simulink model "CruiseControl_pp"  (R2018b)
settings: Solver=ode3  StartTime=0.0  StopTime=16  FixedStep=0.1  RelTol=1e-3  EnableMultiTasking=on
PreLoadFcn:
  | CruiseControl_dd;
  | definePPenums;
undefined symbols (not defined in the file or in its folder): mintspeed
libraries: sldvlib x20, simulink x7
settings Model: SnapshotInterval=1  Creator=The MathWorks Inc.  LastModifiedBy=colosky
settings DataIOCC: LimitDataPoints=on  SaveFormat=Array  SaveOutput=off  SaveTime=off
settings OptimizationCC: DefaultParameterBehavior=Inlined  InlineInvariantSignals=on  ExpressionDepthLimit=2147483647  InitFltsAndDblsToZero=on  LifeSpan=1
settings DebuggingCC: SaveWithParameterizedLinksMsg=none  UnderspecifiedInitializationDetection=Classic  MergeDetectMultiDrivingBlocksExec=none  SolverPrmCheckMsg=warning  FcnCallInpInsideContextMsg=warning  AllowSymbolicDim=off  StateNameClashWarn=warning  LibraryContextMissingDiagnostic=none  StrictBusMsg=ErrorOnBusTreatedAsVector  SFUnexpectedBacktrackingDiag=warning  SFNoUnconditionalDefaultTransitionDiag=warning  SFExecutionAtInitializationDiag=none
settings HardwareCC: ProdBitPerPointer=32  ProdBitPerSizeT=32  ProdBitPerPtrDiffT=32  ProdLargestAtomicFloat=None  ProdEndianess=Unspecified  ProdWordSize=32  ProdHWDeviceType=32-bit Generic
settings ModelReferenceCC: ModelReferenceNumInstancesAllowed=Single  PropagateSignalLabelsOutOfModel=off
settings SFSimCC: SimUseLocalCustomCode=off  SimParseCustomCode=off  MATLABDynamicMemAlloc=off
settings RTWCC: SystemTargetFile=ert.tlc  TemplateMakefile=ert_default_tmf  GenerateReport=on  RTWUseLocalCustomCode=off  IncludeHyperlinkInReport=on  LaunchReport=on  GenerateTraceInfo=on  GenerateTraceReport=on  GenerateTraceReportSl=on  GenerateTraceReportSf=on  GenerateTraceReportEml=on
settings CodeAppCC: ForceParamTrailComments=on  IgnoreCustomStorageClasses=off  OperatorAnnotations=on  SimulinkDataObjDesc=on  SFDataObjDesc=on  MATLABFcnDesc=on  InsertBlockDesc=on  StateflowObjectComments=on  MATLABSourceComments=on
settings ERTTargetCC: MultiwordLength=2048  GenerateSampleERTMain=on  InlinedParameterPlacement=NonHierarchical  ERTCustomFileTemplate=example_file_process.tlc
settings ConfigComp: CovEnable=on  CovScope=ReferencedModels  RecordCoverage=on  CovMetricSettings=dcme  CovModelRefEnable=Off  CovExternalEMLEnable=off  CovSFcnEnable=off  DVMode=PropertyProving  DVMaxProcessTime=3000  DVDisplayUnsatisfiableObjectives=on  DVAutomaticStubbing=off  DVMakeOutputFilesUnique=off  DVModelCoverageObjectives=MCDC  DVMaxTestCaseSteps=500  DVTestSuiteOptimization=CombinedObjectives  DVAssertions=EnableAll  DVProofAssumptions=EnableAll  DVDetectActiveLogic=on  DVDetectIntegerOverflow=off  DVMaxViolationSteps=10  DVSaveDataFile=off  DVSaveHarnessModel=on  DVReportIncludeGraphics=on  DVDisplayResultsOnModel=on

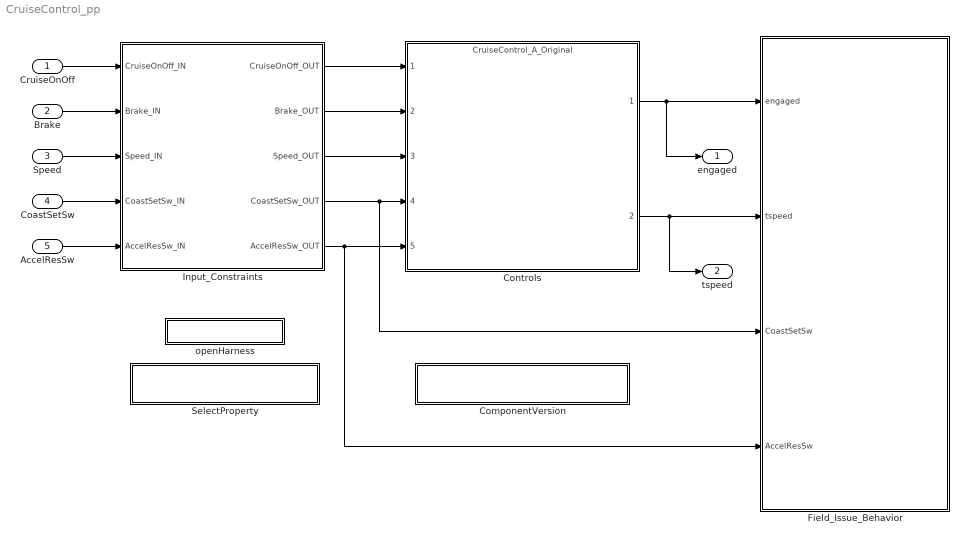
== system CruiseControl_pp ==
  CruiseOnOff : Inport  OutDataTypeStr=boolean  PortDimensions=1
  Brake : Inport  Port=2  OutDataTypeStr=boolean  PortDimensions=1
  Speed : Inport  Port=3  OutDataTypeStr=uint8  PortDimensions=1
  CoastSetSw : Inport  Port=4  OutDataTypeStr=boolean  PortDimensions=1
  AccelResSw : Inport  Port=5  OutDataTypeStr=boolean  PortDimensions=1
  ComponentVersion : Subsystem
      settings: OpenFcn=|
      | [~,enumVers] = enumeration('CtrlsVerEnum');
      | [selection, ok] = listdlg('Name','Component Version','ListSize',[210 110],'SelectionMode','single', ...
      |    'PromptString','Select Cruise Control version...','ListString',enumVers,'InitialValue',uint32(CtrlsVer));
      | waitfor(selection);
      | if ok
      |    CtrlsVer = CtrlsVerEnum(enumVers{selection});
      | end
      mask Display: disp('Select Cruise Control version to verify');
  Controls : ModelReference  ModelNameDialog=CruiseControl_A_Original.slx  SimulationMode=Normal  Variant=on  ModelReferenceVersion=1.516
  Field_Issue_Behavior : Subsystem  Variant=on
      settings: AttributesFormatString=%<BlockChoice>
  Input_Constraints : Subsystem  Variant=on
      settings: AttributesFormatString=%<BlockChoice>
  SelectProperty : Subsystem
      settings: OpenFcn=|
      | [~,enumProps] = enumeration('PropEnum');
      | [selection, ok] = listdlg('Name','Propery To Prove','ListSize',[210 110],'SelectionMode','single', ...
      |    'PromptString','Select Property to Prove...','ListString',enumProps,'InitialValue',uint32(Prop2Prove));
      | waitfor(selection);
      | if ok
      |    Prop2Prove = PropEnum(enumProps{selection});
      | end
      mask Display: disp('Select Property to Prove...');
  openHarness : Subsystem
      settings: OpenFcn=|
      | switch (CtrlsVer)
      | case CtrlsVerEnum.CtrlC_ExecOrder_fix
      |     load_PP_harness('CruiseControl_pp_harness_FieldIssue');
      | case CtrlsVerEnum.CtrlD_ExecOrderSneak_fix
      |     load_PP_harness('CruiseControl_pp_harness_ReqProve');
      | case CtrlsVerEnum.CtrlE_ExecOrderSneakDblReject_fix
      |     load_PP_harness('CruiseControl_pp_harness_ReqWithParsProve');
      | end
      mask Display: disp(['Open Harness']);
  engaged : Outport  OutDataTypeStr=boolean  PortDimensions=1
  tspeed : Outport  Port=2  OutDataTypeStr=uint8  PortDimensions=1
  wires:
  Controls/2 -> tspeed/1, Field_Issue_Behavior/2(tspeed)
  AccelResSw/1 -> Input_Constraints/5(AccelResSw_IN)
  Speed/1 -> Input_Constraints/3(Speed_IN)
  CruiseOnOff/1 -> Input_Constraints/1(CruiseOnOff_IN)
  Brake/1 -> Input_Constraints/2(Brake_IN)
  CoastSetSw/1 -> Input_Constraints/4(CoastSetSw_IN)
  Input_Constraints/1(CruiseOnOff_OUT) -> Controls/1
  Input_Constraints/2(Brake_OUT) -> Controls/2
  Input_Constraints/3(Speed_OUT) -> Controls/3
  Input_Constraints/4(CoastSetSw_OUT) -> Field_Issue_Behavior/3(CoastSetSw), Controls/4
  Input_Constraints/5(AccelResSw_OUT) -> Field_Issue_Behavior/4(AccelResSw), Controls/5
  Controls/1 -> engaged/1, Field_Issue_Behavior/1(engaged)

== system CruiseControl_pp/ComponentVersion ==

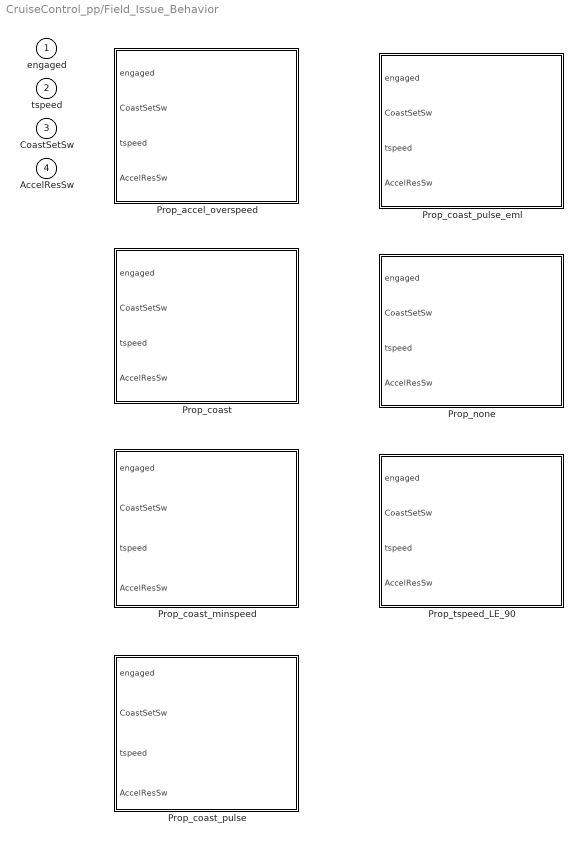
== system CruiseControl_pp/Field_Issue_Behavior ==
  engaged : Inport
  tspeed : Inport  Port=2
  CoastSetSw : Inport  Port=3
  AccelResSw : Inport  Port=4
  Prop_accel_overspeed : Subsystem  VariantControl=Prop2Prove == PropEnum.Prop_accel_overspeed
  Prop_coast : Subsystem  VariantControl=Prop2Prove == PropEnum.Prop_coast
  Prop_coast_minspeed : Subsystem  VariantControl=Prop2Prove == PropEnum.Prop_coast_minspeed
  Prop_coast_pulse : Subsystem  VariantControl=Prop2Prove == PropEnum.Prop_coast_pulse
  Prop_coast_pulse_eml : Subsystem  VariantControl=Prop2Prove == PropEnum.Prop_coast_pulse_eml
  Prop_none : Subsystem  VariantControl=Prop2Prove == PropEnum.Prop_none
  Prop_tspeed_LE_90 : Subsystem  VariantControl=Prop2Prove == PropEnum.Prop_tspeed_LE_90

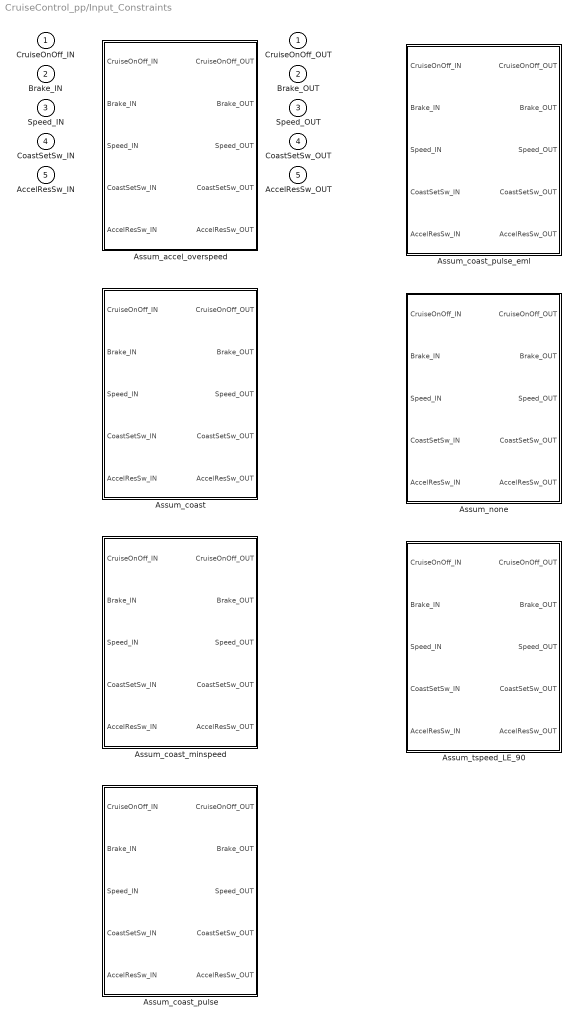
== system CruiseControl_pp/Input_Constraints ==
  CruiseOnOff_IN : Inport
  Brake_IN : Inport  Port=2
  Speed_IN : Inport  Port=3
  CoastSetSw_IN : Inport  Port=4
  AccelResSw_IN : Inport  Port=5
  Assum_accel_overspeed : Subsystem  VariantControl=Prop2Prove == PropEnum.Prop_accel_overspeed
  Assum_coast : Subsystem  VariantControl=Prop2Prove == PropEnum.Prop_coast
  Assum_coast_minspeed : Subsystem  VariantControl=Prop2Prove == PropEnum.Prop_coast_minspeed
  Assum_coast_pulse : Subsystem  VariantControl=Prop2Prove == PropEnum.Prop_coast_pulse
  Assum_coast_pulse_eml : Subsystem  VariantControl=Prop2Prove == PropEnum.Prop_coast_pulse_eml
  Assum_none : Subsystem  VariantControl=Prop2Prove == PropEnum.Prop_none
  Assum_tspeed_LE_90 : Subsystem  VariantControl=Prop2Prove == PropEnum.Prop_tspeed_LE_90
  CruiseOnOff_OUT : Outport
  Brake_OUT : Outport  Port=2
  Speed_OUT : Outport  Port=3
  CoastSetSw_OUT : Outport  Port=4
  AccelResSw_OUT : Outport  Port=5

== system CruiseControl_pp/SelectProperty ==

== system CruiseControl_pp/openHarness ==

== system CruiseControl_pp/Field_Issue_Behavior/Prop_accel_overspeed ==
  engaged : Inport
  CoastSetSw : Inport  Port=2
  tspeed : Inport  Port=3
  AccelResSw : Inport  Port=4
  Compare To Constant : simulink/Logic and Bit Operations/Compare To Constant  relop=<=  const=95  OutDataTypeStr=boolean
  EngagedImplies : sldvlib/Verification Utilities/Implies
      settings: SourceProductName=Simulink Design Verifier  SourceProductBaseCode=DV
  Logical Operator2 : Logic  AllPortsSameDT=off  OutDataTypeStr=boolean
  Prop_accel_overspeed : sldvlib/Objectives and Constraints/Proof Objective  enabled=on  customAVTBlockType=Proof Objective  intervals=true  dispValues=on  outEnabled=off  enableStopSim=off
      settings: AttributesFormatString=%<intervals>  SourceProductName=Simulink Design Verifier  SourceProductBaseCode=DV
  Terminator1 : Terminator
  wires:
  CoastSetSw/1 -> Terminator1/1
  tspeed/1 -> Compare To Constant/1
  Compare To Constant/1 -> EngagedImplies/2
  engaged/1 -> Logical Operator2/1
  AccelResSw/1 -> Logical Operator2/2
  Logical Operator2/1 -> EngagedImplies/1
  EngagedImplies/1 -> Prop_accel_overspeed/1

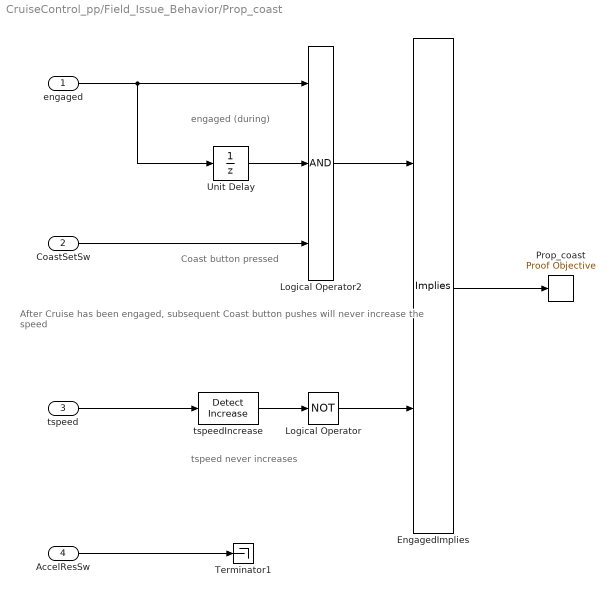
== system CruiseControl_pp/Field_Issue_Behavior/Prop_coast ==
  note: engaged (during)
  note: tspeed never increases
  note: Coast button pressed
  note: After Cruise has been engaged, subsequent Coast button pushes will never increase the speed
  engaged : Inport
  CoastSetSw : Inport  Port=2
  tspeed : Inport  Port=3
  AccelResSw : Inport  Port=4
  EngagedImplies : sldvlib/Verification Utilities/Implies
      settings: SourceProductName=Simulink Design Verifier  SourceProductBaseCode=DV
  Logical Operator : Logic  Operator=NOT  AllPortsSameDT=off  OutDataTypeStr=boolean
  Logical Operator2 : Logic  Inputs=3  AllPortsSameDT=off  OutDataTypeStr=boolean
  Prop_coast : sldvlib/Objectives and Constraints/Proof Objective  enabled=on  customAVTBlockType=Proof Objective  intervals=true  dispValues=on  outEnabled=off  enableStopSim=off
      settings: AttributesFormatString=%<intervals>  SourceProductName=Simulink Design Verifier  SourceProductBaseCode=DV
  Terminator1 : Terminator
  Unit Delay : UnitDelay  SampleTime=-1
  tspeedIncrease : simulink/Logic and Bit Operations/Detect Increase  vinit=0.0  InputProcessing=Inherited  OutDataTypeStr=boolean
  wires:
  Logical Operator2/1 -> EngagedImplies/1
  CoastSetSw/1 -> Logical Operator2/3
  Logical Operator/1 -> EngagedImplies/2
  engaged/1 -> Unit Delay/1, Logical Operator2/1
  AccelResSw/1 -> Terminator1/1
  Unit Delay/1 -> Logical Operator2/2
  tspeed/1 -> tspeedIncrease/1
  tspeedIncrease/1 -> Logical Operator/1
  EngagedImplies/1 -> Prop_coast/1

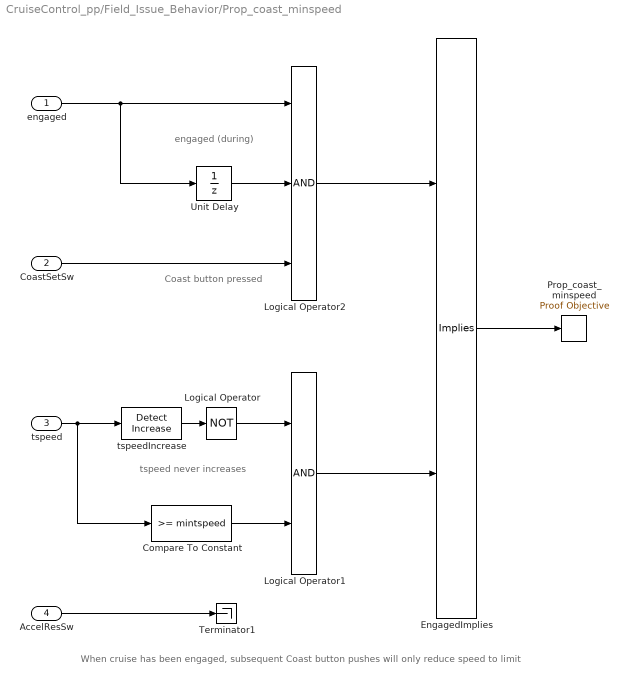
== system CruiseControl_pp/Field_Issue_Behavior/Prop_coast_minspeed ==
  note: engaged (during)
  note: tspeed never increases
  note: Coast button pressed
  note: When cruise has been engaged, subsequent Coast button pushes will only reduce speed to limit
  engaged : Inport
  CoastSetSw : Inport  Port=2
  tspeed : Inport  Port=3
  AccelResSw : Inport  Port=4
  Compare To Constant : simulink/Logic and Bit Operations/Compare To Constant  relop=>=  const=mintspeed  OutDataTypeStr=boolean
  EngagedImplies : sldvlib/Verification Utilities/Implies
      settings: SourceProductName=Simulink Design Verifier  SourceProductBaseCode=DV
  Logical Operator : Logic  Operator=NOT  AllPortsSameDT=off  OutDataTypeStr=boolean
  Logical Operator1 : Logic  AllPortsSameDT=off  OutDataTypeStr=boolean
  Logical Operator2 : Logic  Inputs=3  AllPortsSameDT=off  OutDataTypeStr=boolean
  Prop_coast_minspeed : sldvlib/Objectives and Constraints/Proof Objective  enabled=on  customAVTBlockType=Proof Objective  intervals=true  dispValues=on  outEnabled=off  enableStopSim=off
      settings: AttributesFormatString=%<intervals>  SourceProductName=Simulink Design Verifier  SourceProductBaseCode=DV
  Terminator1 : Terminator
  Unit Delay : UnitDelay  SampleTime=-1
  tspeedIncrease : simulink/Logic and Bit Operations/Detect Increase  vinit=0.0  InputProcessing=Inherited  OutDataTypeStr=boolean
  wires:
  Logical Operator2/1 -> EngagedImplies/1
  CoastSetSw/1 -> Logical Operator2/3
  engaged/1 -> Unit Delay/1, Logical Operator2/1
  AccelResSw/1 -> Terminator1/1
  Unit Delay/1 -> Logical Operator2/2
  tspeed/1 -> Compare To Constant/1, tspeedIncrease/1
  tspeedIncrease/1 -> Logical Operator/1
  EngagedImplies/1 -> Prop_coast_minspeed/1
  Logical Operator/1 -> Logical Operator1/1
  Compare To Constant/1 -> Logical Operator1/2
  Logical Operator1/1 -> EngagedImplies/2

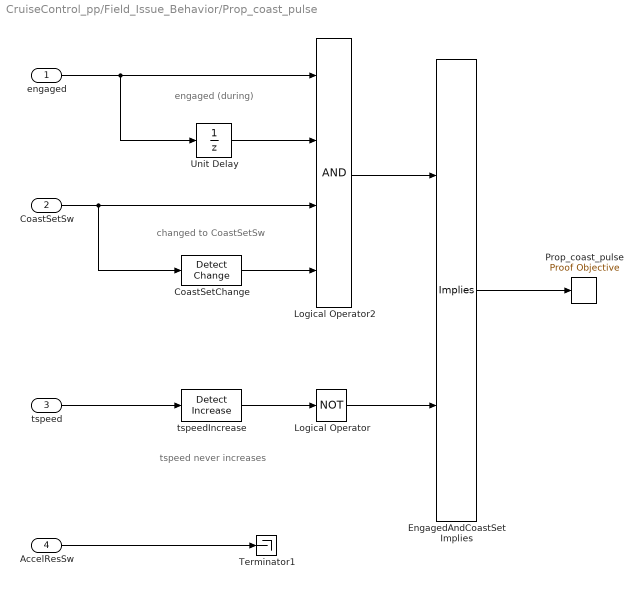
== system CruiseControl_pp/Field_Issue_Behavior/Prop_coast_pulse ==
  note: changed to CoastSetSw
  note: tspeed never increases
  note: engaged (during)
  engaged : Inport
  CoastSetSw : Inport  Port=2
  tspeed : Inport  Port=3
  AccelResSw : Inport  Port=4
  CoastSetChange : simulink/Logic and Bit Operations/Detect Change  vinit=0  OutDataTypeStr=boolean
  EngagedAndCoastSetImplies : sldvlib/Verification Utilities/Implies
      settings: SourceProductName=Simulink Design Verifier  SourceProductBaseCode=DV
  Logical Operator : Logic  Operator=NOT  AllPortsSameDT=off  OutDataTypeStr=boolean
  Logical Operator2 : Logic  Inputs=4  AllPortsSameDT=off  OutDataTypeStr=boolean
  Prop_coast_pulse : sldvlib/Objectives and Constraints/Proof Objective  enabled=on  customAVTBlockType=Proof Objective  intervals=true  dispValues=on  outEnabled=off  enableStopSim=off
      settings: AttributesFormatString=%<intervals>  SourceProductName=Simulink Design Verifier  SourceProductBaseCode=DV
  Terminator1 : Terminator
  Unit Delay : UnitDelay  SampleTime=-1
  tspeedIncrease : simulink/Logic and Bit Operations/Detect Increase  vinit=0.0  InputProcessing=Inherited  OutDataTypeStr=boolean
  wires:
  Logical Operator/1 -> EngagedAndCoastSetImplies/2
  CoastSetSw/1 -> Logical Operator2/3, CoastSetChange/1
  tspeed/1 -> tspeedIncrease/1
  Logical Operator2/1 -> EngagedAndCoastSetImplies/1
  AccelResSw/1 -> Terminator1/1
  tspeedIncrease/1 -> Logical Operator/1
  EngagedAndCoastSetImplies/1 -> Prop_coast_pulse/1
  engaged/1 -> Unit Delay/1, Logical Operator2/1
  Unit Delay/1 -> Logical Operator2/2
  CoastSetChange/1 -> Logical Operator2/4

== system CruiseControl_pp/Field_Issue_Behavior/Prop_coast_pulse_eml ==
  engaged : Inport
  CoastSetSw : Inport  Port=2
  tspeed : Inport  Port=3
  AccelResSw : Inport  Port=4
  MATLAB Function : Subsystem  TreatAsAtomicUnit=on
  Porp_coast_pulse_eml : sldvlib/Objectives and Constraints/Proof Objective  enabled=on  customAVTBlockType=Proof Objective  intervals=true  dispValues=on  outEnabled=off  enableStopSim=off
      settings: AttributesFormatString=%<intervals>  SourceProductName=Simulink Design Verifier  SourceProductBaseCode=DV
  Terminator1 : Terminator
  wires:
  AccelResSw/1 -> Terminator1/1
  engaged/1 -> MATLAB Function/1(engaged)
  CoastSetSw/1 -> MATLAB Function/2(CoastSetSw)
  tspeed/1 -> MATLAB Function/3(tspeed)
  MATLAB Function/1(property) -> Porp_coast_pulse_eml/1

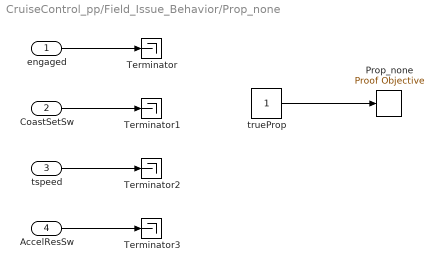
== system CruiseControl_pp/Field_Issue_Behavior/Prop_none ==
  engaged : Inport
  CoastSetSw : Inport  Port=2
  tspeed : Inport  Port=3
  AccelResSw : Inport  Port=4
  Prop_none : sldvlib/Objectives and Constraints/Proof Objective  enabled=on  customAVTBlockType=Proof Objective  intervals=true  dispValues=on  outEnabled=off  enableStopSim=off
      settings: AttributesFormatString=%<intervals>  SourceProductName=Simulink Design Verifier  SourceProductBaseCode=DV
  Terminator{,1..3} (4 alike) : Terminator
  trueProp : Constant  OutDataTypeStr=boolean
  wires:
  CoastSetSw/1 -> Terminator1/1
  tspeed/1 -> Terminator2/1
  engaged/1 -> Terminator/1
  AccelResSw/1 -> Terminator3/1
  trueProp/1 -> Prop_none/1

== system CruiseControl_pp/Field_Issue_Behavior/Prop_tspeed_LE_90 ==
  engaged : Inport
  CoastSetSw : Inport  Port=2
  tspeed : Inport  Port=3
  AccelResSw : Inport  Port=4
  Compare To Constant : simulink/Logic and Bit Operations/Compare To Constant  relop=<=  const=90  OutDataTypeStr=boolean
  Prop_tspeed_LE_90 : sldvlib/Objectives and Constraints/Proof Objective  enabled=on  customAVTBlockType=Proof Objective  intervals=true  dispValues=on  outEnabled=off  enableStopSim=off
      settings: AttributesFormatString=%<intervals>  SourceProductName=Simulink Design Verifier  SourceProductBaseCode=DV
  Terminator : Terminator
  Terminator1 : Terminator
  Terminator2 : Terminator
  wires:
  engaged/1 -> Terminator/1
  tspeed/1 -> Compare To Constant/1
  CoastSetSw/1 -> Terminator1/1
  AccelResSw/1 -> Terminator2/1
  Compare To Constant/1 -> Prop_tspeed_LE_90/1

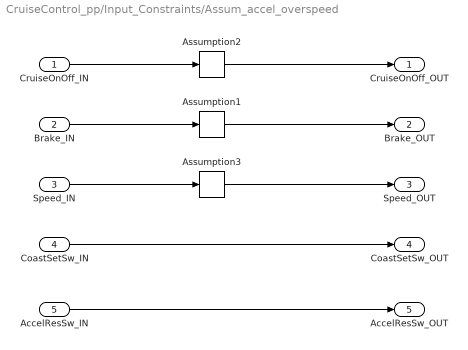
== system CruiseControl_pp/Input_Constraints/Assum_accel_overspeed ==
  CruiseOnOff_IN : Inport  OutDataTypeStr=boolean  PortDimensions=1
  Brake_IN : Inport  Port=2  OutDataTypeStr=boolean  PortDimensions=1
  Speed_IN : Inport  Port=3  OutDataTypeStr=uint8  PortDimensions=1
  CoastSetSw_IN : Inport  Port=4  OutDataTypeStr=boolean  PortDimensions=1
  AccelResSw_IN : Inport  Port=5  OutDataTypeStr=boolean  PortDimensions=1
  Assumption1 : sldvlib/Objectives and Constraints/Assumption  enabled=on  customAVTBlockType=Assumption  intervals=false  initial=off  dispValues=on  outEnabled=on
      settings: AttributesFormatString=%<intervals>  SourceProductName=Simulink Design Verifier  SourceProductBaseCode=DV
  Assumption2 : sldvlib/Objectives and Constraints/Assumption  enabled=on  customAVTBlockType=Assumption  intervals=true  initial=off  dispValues=on  outEnabled=on
      settings: AttributesFormatString=%<intervals>  SourceProductName=Simulink Design Verifier  SourceProductBaseCode=DV
  Assumption3 : sldvlib/Objectives and Constraints/Assumption  enabled=on  customAVTBlockType=Assumption  intervals={[88 Inf]}  initial=off  dispValues=on  outEnabled=on
      settings: AttributesFormatString=%<intervals>  SourceProductName=Simulink Design Verifier  SourceProductBaseCode=DV
  CruiseOnOff_OUT : Outport
  Brake_OUT : Outport  Port=2
  Speed_OUT : Outport  Port=3
  CoastSetSw_OUT : Outport  Port=4
  AccelResSw_OUT : Outport  Port=5
  wires:
  Speed_IN/1 -> Assumption3/1
  CoastSetSw_IN/1 -> CoastSetSw_OUT/1
  AccelResSw_IN/1 -> AccelResSw_OUT/1
  Brake_IN/1 -> Assumption1/1
  CruiseOnOff_IN/1 -> Assumption2/1
  Assumption2/1 -> CruiseOnOff_OUT/1
  Assumption1/1 -> Brake_OUT/1
  Assumption3/1 -> Speed_OUT/1

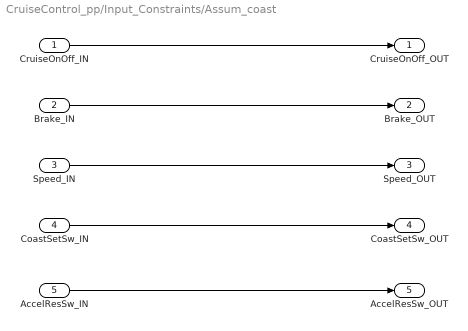
== system CruiseControl_pp/Input_Constraints/Assum_coast ==
  CruiseOnOff_IN : Inport  OutDataTypeStr=boolean  PortDimensions=1
  Brake_IN : Inport  Port=2  OutDataTypeStr=boolean  PortDimensions=1
  Speed_IN : Inport  Port=3  OutDataTypeStr=uint8  PortDimensions=1
  CoastSetSw_IN : Inport  Port=4  OutDataTypeStr=boolean  PortDimensions=1
  AccelResSw_IN : Inport  Port=5  OutDataTypeStr=boolean  PortDimensions=1
  CruiseOnOff_OUT : Outport
  Brake_OUT : Outport  Port=2
  Speed_OUT : Outport  Port=3
  CoastSetSw_OUT : Outport  Port=4
  AccelResSw_OUT : Outport  Port=5
  wires:
  CoastSetSw_IN/1 -> CoastSetSw_OUT/1
  Speed_IN/1 -> Speed_OUT/1
  CruiseOnOff_IN/1 -> CruiseOnOff_OUT/1
  Brake_IN/1 -> Brake_OUT/1
  AccelResSw_IN/1 -> AccelResSw_OUT/1

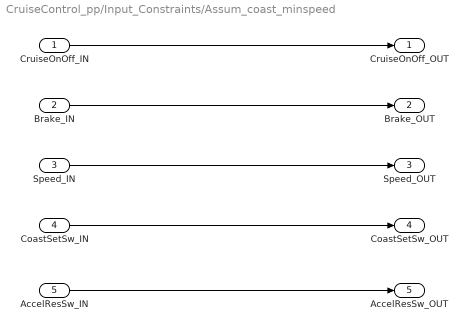
== system CruiseControl_pp/Input_Constraints/Assum_coast_minspeed ==
  CruiseOnOff_IN : Inport  OutDataTypeStr=boolean  PortDimensions=1
  Brake_IN : Inport  Port=2  OutDataTypeStr=boolean  PortDimensions=1
  Speed_IN : Inport  Port=3  OutDataTypeStr=uint8  PortDimensions=1
  CoastSetSw_IN : Inport  Port=4  OutDataTypeStr=boolean  PortDimensions=1
  AccelResSw_IN : Inport  Port=5  OutDataTypeStr=boolean  PortDimensions=1
  CruiseOnOff_OUT : Outport
  Brake_OUT : Outport  Port=2
  Speed_OUT : Outport  Port=3
  CoastSetSw_OUT : Outport  Port=4
  AccelResSw_OUT : Outport  Port=5
  wires:
  CoastSetSw_IN/1 -> CoastSetSw_OUT/1
  Speed_IN/1 -> Speed_OUT/1
  CruiseOnOff_IN/1 -> CruiseOnOff_OUT/1
  Brake_IN/1 -> Brake_OUT/1
  AccelResSw_IN/1 -> AccelResSw_OUT/1

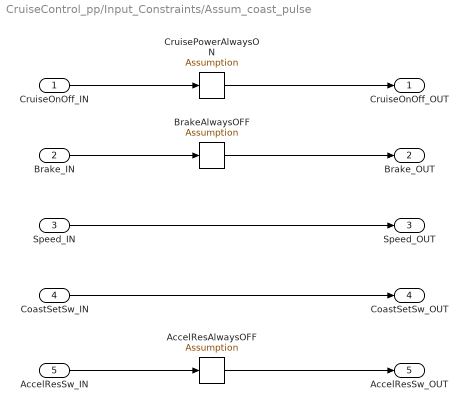
== system CruiseControl_pp/Input_Constraints/Assum_coast_pulse ==
  CruiseOnOff_IN : Inport  OutDataTypeStr=boolean  PortDimensions=1
  Brake_IN : Inport  Port=2  OutDataTypeStr=boolean  PortDimensions=1
  Speed_IN : Inport  Port=3  OutDataTypeStr=uint8  PortDimensions=1
  CoastSetSw_IN : Inport  Port=4  OutDataTypeStr=boolean  PortDimensions=1
  AccelResSw_IN : Inport  Port=5  OutDataTypeStr=boolean  PortDimensions=1
  AccelResAlwaysOFF : sldvlib/Objectives and Constraints/Assumption  enabled=on  customAVTBlockType=Assumption  intervals=false  initial=off  dispValues=on  outEnabled=on
      settings: AttributesFormatString=%<intervals>  SourceProductName=Simulink Design Verifier  SourceProductBaseCode=DV
  BrakeAlwaysOFF : sldvlib/Objectives and Constraints/Assumption  enabled=on  customAVTBlockType=Assumption  intervals=false  initial=off  dispValues=on  outEnabled=on
      settings: AttributesFormatString=%<intervals>  SourceProductName=Simulink Design Verifier  SourceProductBaseCode=DV
  CruisePowerAlwaysON : sldvlib/Objectives and Constraints/Assumption  enabled=on  customAVTBlockType=Assumption  intervals=true  initial=off  dispValues=on  outEnabled=on
      settings: AttributesFormatString=%<intervals>  SourceProductName=Simulink Design Verifier  SourceProductBaseCode=DV
  CruiseOnOff_OUT : Outport
  Brake_OUT : Outport  Port=2
  Speed_OUT : Outport  Port=3
  CoastSetSw_OUT : Outport  Port=4
  AccelResSw_OUT : Outport  Port=5
  wires:
  AccelResAlwaysOFF/1 -> AccelResSw_OUT/1
  BrakeAlwaysOFF/1 -> Brake_OUT/1
  CruisePowerAlwaysON/1 -> CruiseOnOff_OUT/1
  CruiseOnOff_IN/1 -> CruisePowerAlwaysON/1
  Brake_IN/1 -> BrakeAlwaysOFF/1
  Speed_IN/1 -> Speed_OUT/1
  AccelResSw_IN/1 -> AccelResAlwaysOFF/1
  CoastSetSw_IN/1 -> CoastSetSw_OUT/1

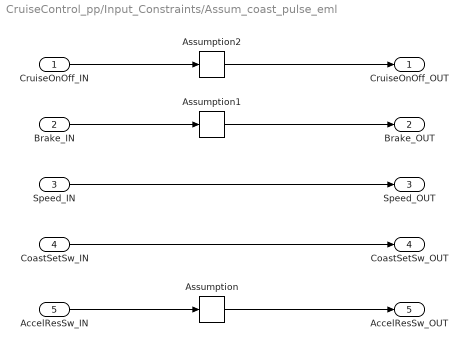
== system CruiseControl_pp/Input_Constraints/Assum_coast_pulse_eml ==
  CruiseOnOff_IN : Inport  OutDataTypeStr=boolean  PortDimensions=1
  Brake_IN : Inport  Port=2  OutDataTypeStr=boolean  PortDimensions=1
  Speed_IN : Inport  Port=3  OutDataTypeStr=uint8  PortDimensions=1
  CoastSetSw_IN : Inport  Port=4  OutDataTypeStr=boolean  PortDimensions=1
  AccelResSw_IN : Inport  Port=5  OutDataTypeStr=boolean  PortDimensions=1
  Assumption : sldvlib/Objectives and Constraints/Assumption  enabled=on  customAVTBlockType=Assumption  intervals=false  initial=off  dispValues=on  outEnabled=on
      settings: AttributesFormatString=%<intervals>  SourceProductName=Simulink Design Verifier  SourceProductBaseCode=DV
  Assumption1 : sldvlib/Objectives and Constraints/Assumption  enabled=on  customAVTBlockType=Assumption  intervals=false  initial=off  dispValues=on  outEnabled=on
      settings: AttributesFormatString=%<intervals>  SourceProductName=Simulink Design Verifier  SourceProductBaseCode=DV
  Assumption2 : sldvlib/Objectives and Constraints/Assumption  enabled=on  customAVTBlockType=Assumption  intervals=true  initial=off  dispValues=on  outEnabled=on
      settings: AttributesFormatString=%<intervals>  SourceProductName=Simulink Design Verifier  SourceProductBaseCode=DV
  CruiseOnOff_OUT : Outport
  Brake_OUT : Outport  Port=2
  Speed_OUT : Outport  Port=3
  CoastSetSw_OUT : Outport  Port=4
  AccelResSw_OUT : Outport  Port=5
  wires:
  CoastSetSw_IN/1 -> CoastSetSw_OUT/1
  AccelResSw_IN/1 -> Assumption/1
  Speed_IN/1 -> Speed_OUT/1
  Brake_IN/1 -> Assumption1/1
  CruiseOnOff_IN/1 -> Assumption2/1
  Assumption2/1 -> CruiseOnOff_OUT/1
  Assumption1/1 -> Brake_OUT/1
  Assumption/1 -> AccelResSw_OUT/1

== system CruiseControl_pp/Input_Constraints/Assum_none ==
  CruiseOnOff_IN : Inport  OutDataTypeStr=boolean  PortDimensions=1
  Brake_IN : Inport  Port=2  OutDataTypeStr=boolean  PortDimensions=1
  Speed_IN : Inport  Port=3  OutDataTypeStr=uint8  PortDimensions=1
  CoastSetSw_IN : Inport  Port=4  OutDataTypeStr=boolean  PortDimensions=1
  AccelResSw_IN : Inport  Port=5  OutDataTypeStr=boolean  PortDimensions=1
  CruiseOnOff_OUT : Outport
  Brake_OUT : Outport  Port=2
  Speed_OUT : Outport  Port=3
  CoastSetSw_OUT : Outport  Port=4
  AccelResSw_OUT : Outport  Port=5
  wires:
  CoastSetSw_IN/1 -> CoastSetSw_OUT/1
  AccelResSw_IN/1 -> AccelResSw_OUT/1
  Speed_IN/1 -> Speed_OUT/1
  Brake_IN/1 -> Brake_OUT/1
  CruiseOnOff_IN/1 -> CruiseOnOff_OUT/1

== system CruiseControl_pp/Input_Constraints/Assum_tspeed_LE_90 ==
  CruiseOnOff_IN : Inport  OutDataTypeStr=boolean  PortDimensions=1
  Brake_IN : Inport  Port=2  OutDataTypeStr=boolean  PortDimensions=1
  Speed_IN : Inport  Port=3  OutDataTypeStr=uint8  PortDimensions=1
  CoastSetSw_IN : Inport  Port=4  OutDataTypeStr=boolean  PortDimensions=1
  AccelResSw_IN : Inport  Port=5  OutDataTypeStr=boolean  PortDimensions=1
  CruiseOnOff_OUT : Outport
  Brake_OUT : Outport  Port=2
  Speed_OUT : Outport  Port=3
  CoastSetSw_OUT : Outport  Port=4
  AccelResSw_OUT : Outport  Port=5
  wires:
  CruiseOnOff_IN/1 -> CruiseOnOff_OUT/1
  Brake_IN/1 -> Brake_OUT/1
  AccelResSw_IN/1 -> AccelResSw_OUT/1
  CoastSetSw_IN/1 -> CoastSetSw_OUT/1
  Speed_IN/1 -> Speed_OUT/1

== system CruiseControl_pp/Field_Issue_Behavior/Prop_coast_pulse_eml/MATLAB Function ==
  engaged : Inport
  CoastSetSw : Inport  Port=2
  tspeed : Inport  Port=3
  " Demux " : Demux  Outputs=1
  " SFunction " : S-Function  Tag=Stateflow S-Function propertyLib 2  FunctionName=sf_sfun  PortCounts=[3 2]  SFunctionDeploymentMode=off  EnableBusSupport=off
  " Terminator " : Terminator
  property : Outport
  wires:
  engaged/1 -> " SFunction "/1
  CoastSetSw/1 -> " SFunction "/2
  tspeed/1 -> " SFunction "/3
  " SFunction "/2 -> property/1  "property"
  " Demux "/1 -> " Terminator "/1
  " SFunction "/1 -> " Demux "/1
